simulink model "Demo_CooperativeDriving_cs"  (Simulink 7.6)
settings: Solver=ode5  SolverMode=SingleTasking  StartTime=0.0  StopTime=8  FixedStep=1/20  RelTol=1e-3
PreLoadFcn:
  | check_NUTS_defined
  | model_closed = 0;
  | assignin('base',['model_closed_' bdroot],false);
InitFcn:
  | PreScanExperimentInitFcn(bdroot)
StopFcn:
  | PreScanExperimentStopFcn(bdroot);
  | 
values from neighbouring files (symbols this model uses):
  Cf = (MLV+MRV)*g/2    (= 5460.246)    [shared_pars.m]
  Cr = (MLA+MRA)*g/2    (= 3937.734)    [shared_pars.m]
  Jzz = J_zz + 2*m_wheel*lva^2 + 2*m_wheel*laa^2    (= 3255.36268364)    [shared_pars.m]
  Kaa = 200000    [shared_pars.m]
  Kf = Kva/(g*(MLV+MRV))    (= 18.3141931701)    [shared_pars.m]
  Kr = Kaa/(g*(MLA+MRA))    (= 25.3953161895)    [shared_pars.m]
  Kva = 200000    [shared_pars.m]
  laa = l - lva    (= 1.67328601253)    [shared_pars.m]
  lva = l*(MLA+MRA)/m    (= 1.20671398747)    [shared_pars.m]
  m = MLV+MRV+MLA+MRA    (= 1916)    [shared_pars.m]
  Mu = 1    [simulinkmodel.m]
  relax_on = 0    [simulinkmodel.m]
  sigma_f = 0.65    [simulinkmodel.m]
  sigma_r = 0.65    [simulinkmodel.m]
  TyreType = 1    [simulinkmodel.m]
undefined symbols (not defined in the file or in its folder): DiscIntNeverNeededParam
libraries: PreScanSimulinkLibrary x14, PreScanUsefulBlocks x6, simulink_extras x5
(part 6 of 6)

== system Demo_CooperativeDriving_cs/Toyota_Previa_1/Swarm Behavior/Vehicle/tyre_forces/tyre_rear/Borstel ==
  alpha : Inport
  Fz : Inport  Port=2
  Mu : Inport  Port=3
  Kt : Inport  Port=4
  Abs : Abs  SaturateOnIntegerOverflow=on
  F : Fcn  Expr=(3*u(2) - 3*u(2)^2 + u(2)^3)*u(1)
  Fmax : Fcn  Expr=u(1)
  Gain : Gain  Gain=1/3  SaturateOnIntegerOverflow=on  OutDataTypeStr=Inherit: Same as input  ParamDataTypeStr=Inherit: Same as input
  Math Function : Math  Operator=reciprocal  SaturateOnIntegerOverflow=on
  Mux1 : Mux  Inputs=2
  Product : Product  SaturateOnIntegerOverflow=on  RndMeth=Zero  InputSameDT=on  OutDataTypeStr=Inherit: Same as first input
  Product1 : Product  Inputs=3  SaturateOnIntegerOverflow=on  RndMeth=Zero  InputSameDT=on  OutDataTypeStr=Inherit: Same as first input
  Relational Operator : RelationalOperator  InputSameDT=on
  Sign : Signum
  Switch : Switch  Threshold=0.5  SaturateOnIntegerOverflow=on  InputSameDT=on
  Trigonometric Function : Trigonometry  Operator=tan
  Fy : Outport
  wires:
  Abs/1 -> Relational Operator/1, Product/1
  Kt/1 -> Gain/1
  Relational Operator/1 -> Switch/2
  Trigonometric Function/1 -> Abs/1
  Mux1/1 -> F/1, Fmax/1
  Sign/1 -> Mux1/1
  Product/1 -> Mux1/2
  F/1 -> Switch/3
  Fmax/1 -> Switch/1
  alpha/1 -> Trigonometric Function/1, Sign/1
  Switch/1 -> Product1/1
  Product1/1 -> Fy/1
  Fz/1 -> Product1/2
  Mu/1 -> Product1/3
  Gain/1 -> Product/2, Math Function/1
  Math Function/1 -> Relational Operator/2

== system Demo_CooperativeDriving_cs/Toyota_Previa_1/Swarm Behavior/Vehicle/tyre_forces/tyre_rear/Exponent ==
  alpha : Inport
  Fz : Inport  Port=2
  Mu : Inport  Port=3
  Kt : Inport  Port=4
  Abs : Abs  SaturateOnIntegerOverflow=on
  MuY Front Wheels : Fcn  Expr=(1 - exp(-u(2)*u(1)))
  Mux1 : Mux  Inputs=2
  Product : Product  Inputs=4  SaturateOnIntegerOverflow=on  RndMeth=Zero  InputSameDT=on  OutDataTypeStr=Inherit: Same as first input
  Saturation2 : Saturate  UpperLimit=inf  LowerLimit=1e-9
  Sign : Signum
  Fy : Outport
  wires:
  Abs/1 -> Saturation2/1
  Saturation2/1 -> Mux1/1
  Mux1/1 -> MuY Front Wheels/1
  Kt/1 -> Mux1/2
  Sign/1 -> Product/1
  MuY Front Wheels/1 -> Product/2
  alpha/1 -> Abs/1, Sign/1
  Product/1 -> Fy/1
  Fz/1 -> Product/3
  Mu/1 -> Product/4

== system Demo_CooperativeDriving_cs/Toyota_Yaris_1/Swarm Behavior/Vehicle Dynamics/tyre_forces/tyre_front/Borstel ==
  alpha : Inport
  Fz : Inport  Port=2
  Mu : Inport  Port=3
  Kt : Inport  Port=4
  Abs : Abs  SaturateOnIntegerOverflow=on
  F : Fcn  Expr=(3*u(2) - 3*u(2)^2 + u(2)^3)*u(1)
  Fmax : Fcn  Expr=u(1)
  Gain : Gain  Gain=1/3  SaturateOnIntegerOverflow=on  OutDataTypeStr=Inherit: Same as input  ParamDataTypeStr=Inherit: Same as input
  Math Function : Math  Operator=reciprocal  SaturateOnIntegerOverflow=on
  Mux1 : Mux  Inputs=2
  Product : Product  SaturateOnIntegerOverflow=on  RndMeth=Zero  InputSameDT=on  OutDataTypeStr=Inherit: Same as first input
  Product1 : Product  Inputs=3  SaturateOnIntegerOverflow=on  RndMeth=Zero  InputSameDT=on  OutDataTypeStr=Inherit: Same as first input
  Relational Operator : RelationalOperator  InputSameDT=on
  Sign : Signum
  Switch : Switch  Threshold=0.5  SaturateOnIntegerOverflow=on  InputSameDT=on
  Trigonometric Function : Trigonometry  Operator=tan
  Fy : Outport
  wires:
  Abs/1 -> Relational Operator/1, Product/1
  Kt/1 -> Gain/1
  Relational Operator/1 -> Switch/2
  Trigonometric Function/1 -> Abs/1
  Mux1/1 -> F/1, Fmax/1
  Sign/1 -> Mux1/1
  Product/1 -> Mux1/2
  F/1 -> Switch/3
  Fmax/1 -> Switch/1
  alpha/1 -> Trigonometric Function/1, Sign/1
  Switch/1 -> Product1/1
  Product1/1 -> Fy/1
  Fz/1 -> Product1/2
  Mu/1 -> Product1/3
  Gain/1 -> Product/2, Math Function/1
  Math Function/1 -> Relational Operator/2

== system Demo_CooperativeDriving_cs/Toyota_Yaris_1/Swarm Behavior/Vehicle Dynamics/tyre_forces/tyre_front/Exponent ==
  alpha : Inport
  Fz : Inport  Port=2
  Mu : Inport  Port=3
  Kt : Inport  Port=4
  Abs : Abs  SaturateOnIntegerOverflow=on
  MuY Front Wheels : Fcn  Expr=(1 - exp(-u(2)*u(1)))
  Mux1 : Mux  Inputs=2
  Product : Product  Inputs=4  SaturateOnIntegerOverflow=on  RndMeth=Zero  InputSameDT=on  OutDataTypeStr=Inherit: Same as first input
  Saturation2 : Saturate  UpperLimit=inf  LowerLimit=1e-9
  Sign : Signum
  Fy : Outport
  wires:
  Abs/1 -> Saturation2/1
  Saturation2/1 -> Mux1/1
  Mux1/1 -> MuY Front Wheels/1
  Kt/1 -> Mux1/2
  Sign/1 -> Product/1
  MuY Front Wheels/1 -> Product/2
  alpha/1 -> Abs/1, Sign/1
  Product/1 -> Fy/1
  Fz/1 -> Product/3
  Mu/1 -> Product/4

== system Demo_CooperativeDriving_cs/Toyota_Yaris_1/Swarm Behavior/Vehicle Dynamics/tyre_forces/tyre_rear/Borstel ==
  alpha : Inport
  Fz : Inport  Port=2
  Mu : Inport  Port=3
  Kt : Inport  Port=4
  Abs : Abs  SaturateOnIntegerOverflow=on
  F : Fcn  Expr=(3*u(2) - 3*u(2)^2 + u(2)^3)*u(1)
  Fmax : Fcn  Expr=u(1)
  Gain : Gain  Gain=1/3  SaturateOnIntegerOverflow=on  OutDataTypeStr=Inherit: Same as input  ParamDataTypeStr=Inherit: Same as input
  Math Function : Math  Operator=reciprocal  SaturateOnIntegerOverflow=on
  Mux1 : Mux  Inputs=2
  Product : Product  SaturateOnIntegerOverflow=on  RndMeth=Zero  InputSameDT=on  OutDataTypeStr=Inherit: Same as first input
  Product1 : Product  Inputs=3  SaturateOnIntegerOverflow=on  RndMeth=Zero  InputSameDT=on  OutDataTypeStr=Inherit: Same as first input
  Relational Operator : RelationalOperator  InputSameDT=on
  Sign : Signum
  Switch : Switch  Threshold=0.5  SaturateOnIntegerOverflow=on  InputSameDT=on
  Trigonometric Function : Trigonometry  Operator=tan
  Fy : Outport
  wires:
  Abs/1 -> Relational Operator/1, Product/1
  Kt/1 -> Gain/1
  Relational Operator/1 -> Switch/2
  Trigonometric Function/1 -> Abs/1
  Mux1/1 -> F/1, Fmax/1
  Sign/1 -> Mux1/1
  Product/1 -> Mux1/2
  F/1 -> Switch/3
  Fmax/1 -> Switch/1
  alpha/1 -> Trigonometric Function/1, Sign/1
  Switch/1 -> Product1/1
  Product1/1 -> Fy/1
  Fz/1 -> Product1/2
  Mu/1 -> Product1/3
  Gain/1 -> Product/2, Math Function/1
  Math Function/1 -> Relational Operator/2

== system Demo_CooperativeDriving_cs/Toyota_Yaris_1/Swarm Behavior/Vehicle Dynamics/tyre_forces/tyre_rear/Exponent ==
  alpha : Inport
  Fz : Inport  Port=2
  Mu : Inport  Port=3
  Kt : Inport  Port=4
  Abs : Abs  SaturateOnIntegerOverflow=on
  MuY Front Wheels : Fcn  Expr=(1 - exp(-u(2)*u(1)))
  Mux1 : Mux  Inputs=2
  Product : Product  Inputs=4  SaturateOnIntegerOverflow=on  RndMeth=Zero  InputSameDT=on  OutDataTypeStr=Inherit: Same as first input
  Saturation2 : Saturate  UpperLimit=inf  LowerLimit=1e-9
  Sign : Signum
  Fy : Outport
  wires:
  Abs/1 -> Saturation2/1
  Saturation2/1 -> Mux1/1
  Mux1/1 -> MuY Front Wheels/1
  Kt/1 -> Mux1/2
  Sign/1 -> Product/1
  MuY Front Wheels/1 -> Product/2
  alpha/1 -> Abs/1, Sign/1
  Product/1 -> Fy/1
  Fz/1 -> Product/3
  Mu/1 -> Product/4
